simulink model "Final_quadrotor_linearized_model_lqr"  (R2024a)
settings: Solver=VariableStepAuto  StartTime=0.0  StopTime=10.0  RelTol=1e-3
undefined symbols (not defined in the file): A_aug, B_aug, C_aug, D_aug, disturbance, g_val, Kx, m_val
settings Model: Creator=yufon  LastModifiedBy=yufon

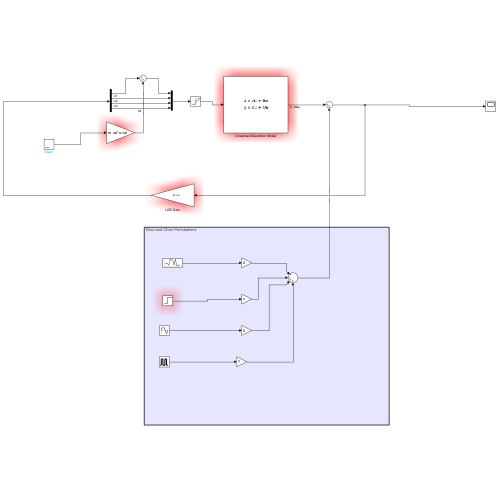
[thumbnail: Simulink's stored preview of the top-level diagram]
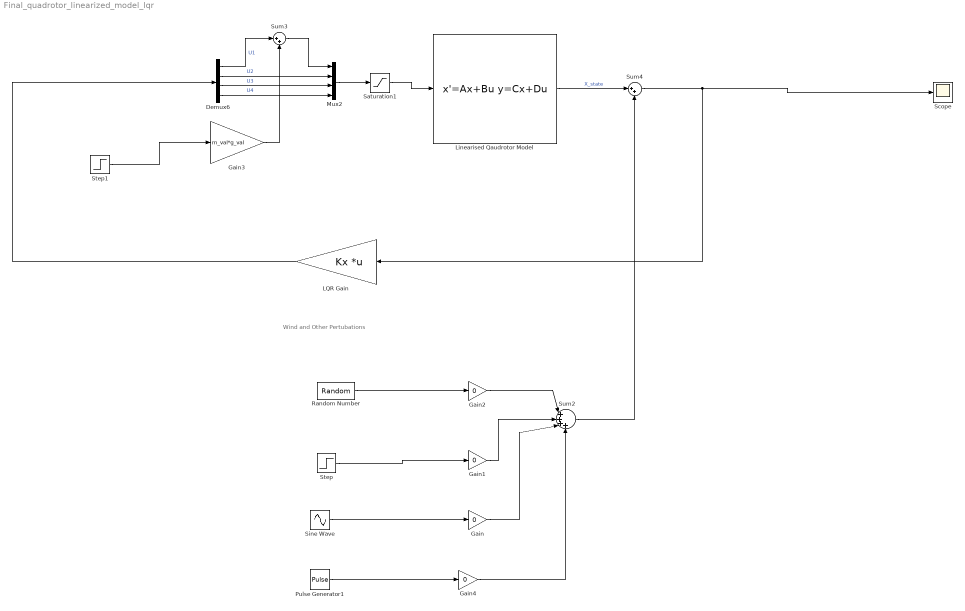
== system Final_quadrotor_linearized_model_lqr ==
  note: Wind and Other Pertubations
  Demux6 : Demux
  Gain{,1..2,4} (4 alike) : Gain  Gain=0
  Gain3 : Gain  Gain=m_val*g_val
  LQR Gain : Gain  Gain=Kx  Multiplication=Matrix(K*u)
  Linearised Qaudrotor Model : StateSpace  A=A_aug  B=B_aug  C=C_aug  D=D_aug  InitialCondition=0
  Mux2 : Mux
  Pulse Generator1 : DiscretePulseGenerator  PulseType=Time based  Period=10  PulseWidth=20  PhaseDelay=5
  Random Number : RandomNumber  Variance=0.5  SampleTime=0.1
  Saturation1 : Saturate  UpperLimit=[30; 0.15; 0.1; 0.5]  LowerLimit=[-3; -0.15; -0.1; -0.5]
  Scope : Scope
  Sine Wave : Sin  Frequency=0.5  SampleTime=0
  Step : Step  Before=zeros(12,1)  After=disturbance  SampleTime=0
  Step1 : Step  Time=10  Before=1  After=1.25  SampleTime=0
  Sum2 : Sum  Inputs=|++++
  Sum3 : Sum  Inputs=|++
  Sum4 : Sum  Inputs=|++
  wires:
  Gain1/1 -> Sum2/2
  Step1/1 -> Gain3/1
  Linearised Qaudrotor Model/1 -> Sum4/1  "X_state"
  LQR Gain/1 -> Demux6/1
  Saturation1/1 -> Linearised Qaudrotor Model/1
  Demux6/2 -> Mux2/2  "U2"
  Gain2/1 -> Sum2/1
  Mux2/1 -> Saturation1/1
  Demux6/3 -> Mux2/3  "U3"
  Demux6/1 -> Sum3/1  "U1"
  Sum3/1 -> Mux2/1
  Sine Wave/1 -> Gain/1
  Random Number/1 -> Gain2/1
  Gain3/1 -> Sum3/2
  Pulse Generator1/1 -> Gain4/1
  Gain/1 -> Sum2/3
  Step/1 -> Gain1/1
  Sum2/1 -> Sum4/2
  Gain4/1 -> Sum2/4
  Demux6/4 -> Mux2/4  "U4"
  Sum4/1 -> LQR Gain/1, Scope/1
